simulink model "kinematik"  (R2025b)
settings: Solver=VariableStepAuto  StartTime=0.0  StopTime=10.0  RelTol=1e-3
undefined symbols (not defined in the file): h0
settings Model: Creator=chris  LastModifiedBy=chris
settings ModelReferenceCC: ModelReferenceMinAlgLoopOccurrences=on

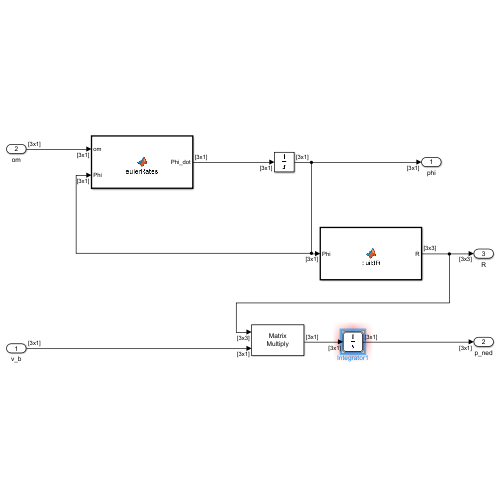
[thumbnail: Simulink's stored preview of the top-level diagram]
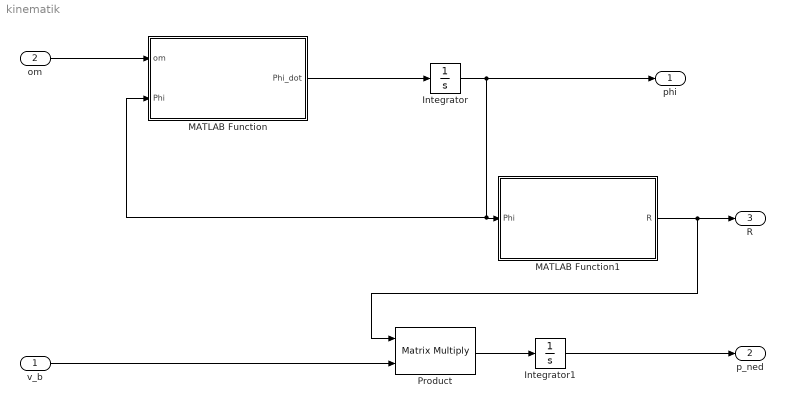
== system kinematik ==
  v_b : Inport  PortDimensions=[3 1]
  om : Inport  Port=2  PortDimensions=[3 1]
  Integrator : Integrator  InitialCondition=[0;0;0]
  Integrator1 : Integrator  InitialCondition=[0;0;h0]
  MATLAB Function : MATLAB Function  TreatAsAtomicUnit=on
  MATLAB Function1 : MATLAB Function  TreatAsAtomicUnit=on
  Product : Product  Multiplication=Matrix(*)
  phi : Outport  PortDimensions=[3 1]
  p_ned : Outport  Port=2
  R : Outport  Port=3  PortDimensions=[3 3]
  wires:
  om/1 -> MATLAB Function/1(om)
  MATLAB Function/1(Phi_dot) -> Integrator/1
  Integrator/1 -> phi/1, MATLAB Function/2(Phi), MATLAB Function1/1(Phi)
  MATLAB Function1/1(R) -> Product/1, R/1
  v_b/1 -> Product/2
  Product/1 -> Integrator1/1
  Integrator1/1 -> p_ned/1

== matlab function kinematik/MATLAB Function ==
  data: om input; Phi_dot output; Phi input
function Phi_dot = eulerRates(om, Phi)
phi = Phi(1); the = Phi(2);
sph=sin(phi); cph=cos(phi); cth=cos(the); tth=tan(the);
W = [1, sph*tth, cph*tth;
     0, cph,    -sph;
     0, sph/cth, cph/cth];   % Singularität bei the = ±pi/2
Phi_dot = W * om;
end

== matlab function kinematik/MATLAB Function1 ==
  data: R output; Phi input
function R = buildR(Phi)
phi=Phi(1); the=Phi(2); psi=Phi(3);
cph=cos(phi); sph=sin(phi); cth=cos(the); sth=sin(the); cps=cos(psi); sps=sin(psi);
R = [cth*cps, sph*sth*cps-cph*sps, cph*sth*cps+sph*sps;
     cth*sps, sph*sth*sps+cph*cps, cph*sth*sps-sph*cps;
    -sth,     sph*cth,             cph*cth];
end
